simulink model "LQG_LQGI"  (R2023b)
settings: Solver=VariableStepAuto  StartTime=0.0  StopTime=10  MaxStep=1e-3  RelTol=1e-3
values from neighbouring files (symbols this model uses):
  A = [0 1;1000 0]    [Parameters.m]
  Bu = [0;20]    [Parameters.m]
  Bw = [1;1]    [Parameters.m]
  C = [1 0]    [Parameters.m]
  N = 1/dcgain(A-Bu*K,Bu,C,0)    [Parameters.m]
undefined symbols (not defined in the file or in its folder): K, Kf, ki
settings Model: Creator=Usuario  LastModifiedBy=JHL
settings SolverCC: AlgebraicLoopSolver=TrustRegion
settings DataIOCC: ReturnWorkspaceOutputs=off
settings DebuggingCC: UnconnectedInputMsg=warning  UnconnectedOutputMsg=warning  UnconnectedLineMsg=warning  ArithmeticOperatorsInVariantConditions=warning
settings ModelReferenceCC: EnableRefExpFcnMdlSchedulingChecks=on
settings SFSimCC: SimUseLocalCustomCode=off  CustomCodeUndefinedFunction=UseInterfaceOnly
settings RTWCC: RTWUseLocalCustomCode=off

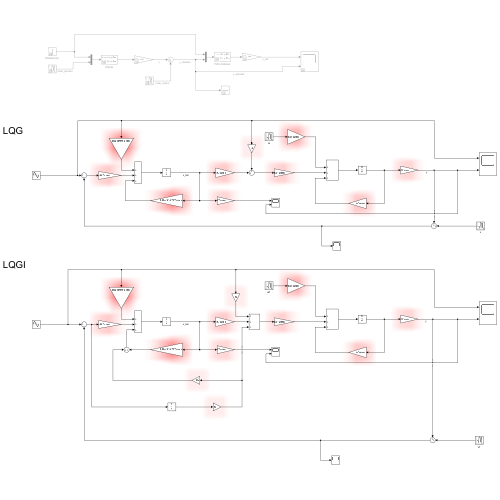
[thumbnail: Simulink's stored preview of the top-level diagram]
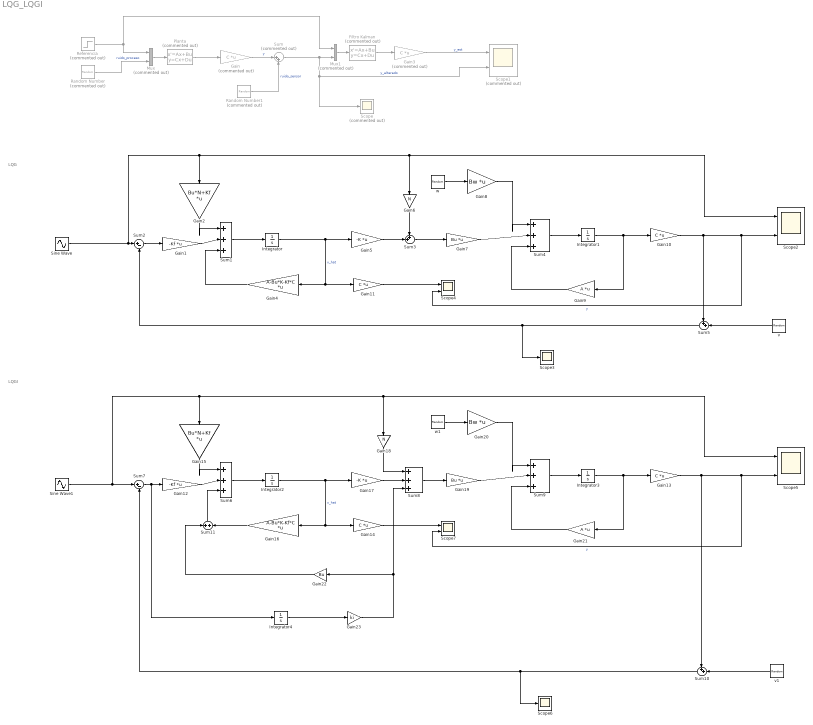
== system LQG_LQGI ==
  note: LQGI
  note: LQG
  "Filtro Kalman " : StateSpace  Commented=on  A=A-Kf*C  B=[Bu Kf]  C=eye(2)  D=zeros(2,2)  InitialCondition=0
  Gain : Gain  Commented=on  Gain=C  Multiplication=Matrix(K*u) (u vector)
  Gain1 : Gain  Gain=-Kf  Multiplication=Matrix(K*u) (u vector)
  Gain{10..11,13..14} (4 alike) : Gain  Gain=C  Multiplication=Matrix(K*u) (u vector)
  Gain12 : Gain  Gain=-Kf  Multiplication=Matrix(K*u) (u vector)
  Gain15 : Gain  Gain=Bu*N+Kf  Multiplication=Matrix(K*u) (u vector)
  Gain16 : Gain  Gain=A-Bu*K-Kf*C  Multiplication=Matrix(K*u) (u vector)
  Gain17 : Gain  Gain=-K  Multiplication=Matrix(K*u) (u vector)
  Gain18 : Gain  Gain=N
  Gain19 : Gain  Gain=Bu  Multiplication=Matrix(K*u) (u vector)
  Gain2 : Gain  Gain=Bu*N+Kf  Multiplication=Matrix(K*u) (u vector)
  Gain20 : Gain  Gain=Bw  Multiplication=Matrix(K*u) (u vector)
  Gain21 : Gain  Gain=A  Multiplication=Matrix(K*u) (u vector)
  Gain22 : Gain  Gain=Bu
  Gain23 : Gain  Gain=ki
  Gain3 : Gain  Commented=on  Gain=C  Multiplication=Matrix(K*u) (u vector)
  Gain4 : Gain  Gain=A-Bu*K-Kf*C  Multiplication=Matrix(K*u) (u vector)
  Gain5 : Gain  Gain=-K  Multiplication=Matrix(K*u) (u vector)
  Gain6 : Gain  Gain=N
  Gain7 : Gain  Gain=Bu  Multiplication=Matrix(K*u) (u vector)
  Gain8 : Gain  Gain=Bw  Multiplication=Matrix(K*u) (u vector)
  Gain9 : Gain  Gain=A  Multiplication=Matrix(K*u) (u vector)
  Integrator{,1..4} (5 alike) : Integrator
  Mux : Mux  Commented=on  Inputs=2
  Mux1 : Mux  Commented=on  Inputs=2
  Planta : StateSpace  Commented=on  A=A  B=[Bu Bw]  C=eye(2)  D=zeros(2,2)  InitialCondition=[1 0]
  Random Number : RandomNumber  Commented=on  Variance=0.2^2  SampleTime=0.01
  Random Number1 : RandomNumber  Commented=on  Variance=0.1^2  SampleTime=0.01  VectorParams1D=off
  Referencia : Step  Commented=on  SampleTime=0
  Scope : Scope  Commented=on
  Scope1 : Scope  Commented=on  NumInputPorts=2
  Scope{2,4..5,7} (4 alike) : Scope  NumInputPorts=2
  Scope3 : Scope
  Scope6 : Scope
  Sine Wave : Sin  Phase=1  SampleTime=0
  Sine Wave1 : Sin  Phase=1  SampleTime=0
  Sum : Sum  Commented=on  Inputs=|++
  Sum{1,4,6,9} (4 alike) : Sum  Inputs=|+++
  Sum10 : Sum  Inputs=++|
  Sum11 : Sum  Inputs=+|+
  Sum2 : Sum  Inputs=|+-
  Sum3 : Sum  Inputs=++|
  Sum5 : Sum  Inputs=++|
  Sum7 : Sum  Inputs=|+-
  Sum8 : Sum  Inputs=+++
  v : RandomNumber  Variance=0.01^2  SampleTime=0.001  VectorParams1D=off
  v1 : RandomNumber  Variance=0.01^2  SampleTime=0.001  VectorParams1D=off
  w : RandomNumber  Variance=0.02^2  SampleTime=0.001
  w1 : RandomNumber  Variance=0.02^2  SampleTime=0.001
  wires:
  Mux1/1 -> "Filtro Kalman "/1
  Sum/1 -> Scope/1, Scope1/2, Mux1/2  "y_alterado"
  Random Number1/1 -> Sum/2  "ruido_sensor"
  Gain/1 -> Sum/1  "y"
  "Filtro Kalman "/1 -> Gain3/1
  Random Number/1 -> Mux/2  "ruido_proceso"
  Planta/1 -> Gain/1
  Mux/1 -> Planta/1
  Referencia/1 -> Mux1/1, Mux/1
  Gain3/1 -> Scope1/1  "y_est"
  Sine Wave/1 -> Scope2/1, Gain6/1, Gain2/1, Sum2/1
  Sum2/1 -> Gain1/1
  Gain1/1 -> Sum1/2
  Gain2/1 -> Sum1/1
  Sum1/1 -> Integrator/1
  Gain4/1 -> Sum1/3
  Integrator/1 -> Gain11/1, Gain4/1, Gain5/1  "x_hat"
  Gain5/1 -> Sum3/2
  Gain6/1 -> Sum3/1
  Sum3/1 -> Gain7/1
  Gain7/1 -> Sum4/2
  w/1 -> Gain8/1
  Gain8/1 -> Sum4/1
  Sum4/1 -> Integrator1/1
  Gain9/1 -> Sum4/3
  Integrator1/1 -> Gain10/1, Gain9/1
  Gain10/1 -> Sum5/1, Scope4/2, Scope2/2  "y"
  v/1 -> Sum5/2
  Sum5/1 -> Scope3/1, Sum2/2
  Gain11/1 -> Scope4/1
  Gain14/1 -> Scope7/1
  Sum10/1 -> Sum7/2, Scope6/1
  v1/1 -> Sum10/2
  Gain13/1 -> Scope5/2, Scope7/2, Sum10/1  "y"
  Integrator3/1 -> Gain21/1, Gain13/1
  Gain21/1 -> Sum9/3
  Sum9/1 -> Integrator3/1
  Gain20/1 -> Sum9/1
  w1/1 -> Gain20/1
  Gain19/1 -> Sum9/2
  Integrator2/1 -> Gain17/1, Gain16/1, Gain14/1  "x_hat"
  Sum6/1 -> Integrator2/1
  Gain15/1 -> Sum6/1
  Gain12/1 -> Sum6/2
  Sum7/1 -> Integrator4/1, Gain12/1
  Sine Wave1/1 -> Sum7/1, Gain15/1, Scope5/1, Gain18/1
  Sum8/1 -> Gain19/1
  Gain17/1 -> Sum8/2
  Gain18/1 -> Sum8/1
  Gain23/1 -> Sum8/3, Gain22/1
  Integrator4/1 -> Gain23/1
  Gain16/1 -> Sum11/2
  Sum11/1 -> Sum6/3
  Gain22/1 -> Sum11/1
